simulink model "cart_phase_control"  (R2013b)
settings: Solver=FixedStepDiscrete  StartTime=0.0  StopTime=4  FixedStep=0.000250  MaxStep=0.5  RelTol=1e-3
InitFcn:
  | % Second Order System Parameters
  | wn = 100;   % Natural Frequency (rad/sec)
  | d  = .4;        % Damping Ratio
libraries: xpclib x5, xpcnilib x2, dspmtrx3 x2, powerlib_meascontrol x1, dspadpt3 x1
Description:
  | This model demonstrates three different representations
  | of a 2nd-Order system.
settings Model: ModifiedHistory="05 Feb 2002  Created."  ExtModeTrigMode=oneshot  ExtModeArmWhenConnect=off  BufferReuse=off  Creator=Douglas G. Jones  LastModifiedBy=bzr3
settings DataIOCC: LimitDataPoints=off  SignalLoggingSaveFormat=ModelDataLogs  SaveOutput=off  SignalLogging=off  SaveTime=off
settings OptimizationCC: BlockReduction=off  BooleanDataType=off  OptimizeBlockIOStorage=off  BufferReuse=off  ExpressionFolding=off  ExpressionDepthLimit=2147483647  LocalBlockOutputs=off  InitFltsAndDblsToZero=on
settings DebuggingCC: SaveWithParameterizedLinksMsg=none  SignalResolutionControl=TryResolveAllWithWarning  SolverPrmCheckMsg=none  MultiTaskDSMMsg=warning  MultiTaskCondExecSysMsg=none  FcnCallInpInsideContextMsg=UseLocalSettings  StateNameClashWarn=warning  StrictBusMsg=None
settings HardwareCC: ProdIntDivRoundTo=Zero  ProdEndianess=LittleEndian  ProdHWDeviceType=Generic->32-bit x86 compatible  TargetLongLongMode=on  TargetEndianess=LittleEndian  TargetHWDeviceType=MATLAB Host
settings RTWCC: SystemTargetFile=xpctarget.tlc  TemplateMakefile=xpc_default_tmf  RTWVerbose=off  ProcessScript=xpctarget_make_rtw_hook  IncludeERTFirstTime=on  RTWCompilerOptimization=On
settings TargetCC: TargetFcnLib=ansi_tfl_tmw.mat  CodeReplacementLibrary=XPC_BLAS  IsPILTarget=off  ParMdlRefBuildCompliant=on  ConcurrentExecutionCompliant=on  MatFileLogging=on  EnableShiftOperators=on
settings ConfigurationSet: Description=SimMechanics 2G

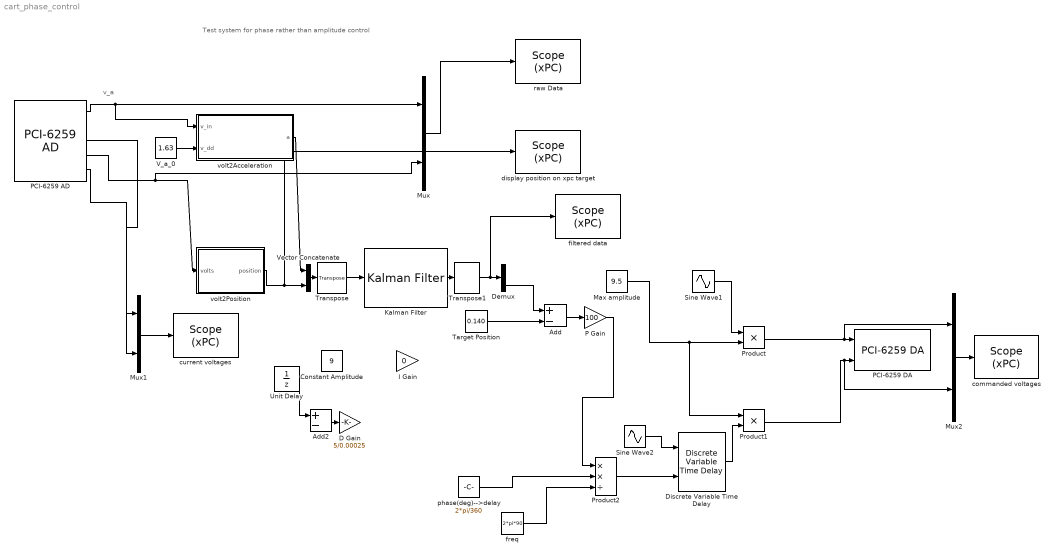
== system cart_phase_control ==
  note: Test system for phase rather than amplitude control
  note: v_a
  Add : Sum  Inputs=+-
  Add2 : Sum  Inputs=+-
  Constant Amplitude : Constant  Value=9
  D Gain : Gain  Gain=5/0.00025
  Demux : Demux  Outputs=2
  Discrete Variable Time Delay : powerlib_meascontrol/Additional Components/Discrete Variable Time Delay  MaxDelay=1  InitialValue=0  Ts=0.00025  DFT=on
  I Gain : Gain  Gain=0
  Kalman Filter : dspadpt3/Kalman Filter  num_targets=1  sourceEnable=Always  isReset=on  X=[0.15;0;0]  P=10*eye(3)  A=[1,2.500000000000000e-04,6.250000000000000e-08;0,1,2.500000000000000e-04;0,0,1]  sourceMeasure=Specify via Dialog  H=[1 0 0; 0 0 1]  Q=0.05*eye(3)  R=[10 0; 0 10]  isOutputEstMeasure=on  isOutputEstState=off  isOutputEstError=off  isOutputPrdMeasure=off  isOutputPrdState=off  isOutputPrdError=off
  Max amplitude : Constant  Value=9.5
  Mux : Mux  Inputs=2
  Mux1 : Mux  Inputs=2
  Mux2 : Mux  Inputs=2
  P Gain : Gain  Gain=100
  PCI-6259 AD : xpcnilib/A//D/M Series/PCI-6259 AD  channel=[1 7 14 16 6]  range=[10]  coupling=[0]  scantime=5e-6  sampletime=0.000250  slot=-1
  PCI-6259 DA : xpcnilib/D//A/M Series/PCI-6259 DA  channel=[1 2]  range=[10]  reset=[1]  initValue=[0]  sampletime=0.00025  slot=-1
  Product : Product  RndMeth=Zero
  Product1 : Product  RndMeth=Zero
  Product2 : Product  Inputs=**/  RndMeth=Zero
  Sine Wave1 : Sin  Frequency=2*pi*90  SampleTime=0
  Sine Wave2 : Sin  Frequency=2*pi*90  Phase=270*pi/180  SampleTime=0
  Target Position : Constant  Value=0.140
  Transpose : dspmtrx3/Transpose  Hermitian=off  overflowFlag=off
  Transpose1 : dspmtrx3/Transpose  Hermitian=off  overflowFlag=off
  Unit Delay : UnitDelay  SampleTime=-1
  V_a_0 : Constant  Value=1.63
  Vector Concatenate : Concatenate  Mode=Multidimensional array  ConcatenateDimension=2
  commanded voltages : xpclib/Misc./Scope (xPC)   scopeno=4  scopetype=Host  autostart=on  viewmode=Graphical redraw  formatstr='%15.6f'  grid=on  ylimits=[0,0]  nosamples=16001  noprepostsamples=0  interleave=1  triggermode=FreeRun  triggersignal=1  trigsignalfromport=off  triggerlevel=0.0  triggerslope=Either  triggerscope=1  triggersample=0  filename=sosLog.dat  mode=Lazy  writesize=512  autorestart=off  dynamicfilemode=off  maxwritefilesize=512*1024^2
  current voltages : xpclib/Misc./Scope (xPC)   scopeno=3  scopetype=Host  autostart=on  viewmode=Graphical redraw  formatstr='%15.6f'  grid=on  ylimits=[0,0]  nosamples=16001  noprepostsamples=0  interleave=1  triggermode=FreeRun  triggersignal=1  trigsignalfromport=off  triggerlevel=0.0  triggerslope=Either  triggerscope=1  triggersample=0  filename=sosLog.dat  mode=Lazy  writesize=512  autorestart=off  dynamicfilemode=off  maxwritefilesize=512*1024^2
  "display position on xpc target " : xpclib/Misc./Scope (xPC)   scopeno=1  scopetype=Target  autostart=on  viewmode=Graphical sliding  formatstr='%15.6f'  grid=on  ylimits=[0,0]  nosamples=16001  noprepostsamples=0  interleave=1  triggermode=FreeRun  triggersignal=1  trigsignalfromport=off  triggerlevel=0.0  triggerslope=Either  triggerscope=1  triggersample=0  filename=sosLog.dat  mode=Lazy  writesize=512  autorestart=off  dynamicfilemode=off  maxwritefilesize=512*1024^2
  filtered data : xpclib/Misc./Scope (xPC)   scopeno=2  scopetype=Host  autostart=on  viewmode=Graphical redraw  formatstr='%15.6f'  grid=on  ylimits=[0,0]  nosamples=16001  noprepostsamples=0  interleave=1  triggermode=FreeRun  triggersignal=1  trigsignalfromport=off  triggerlevel=0.0  triggerslope=Either  triggerscope=1  triggersample=0  filename=sosLog.dat  mode=Lazy  writesize=512  autorestart=off  dynamicfilemode=off  maxwritefilesize=512*1024^2
  freq : Constant  Value=2*pi*90
  phase(deg)-->delay : Constant  Value=2*pi/360
  raw Data : xpclib/Misc./Scope (xPC)   scopeno=5  scopetype=Host  autostart=on  viewmode=Graphical redraw  formatstr='%15.6f'  grid=on  ylimits=[0,0]  nosamples=16001  noprepostsamples=0  interleave=1  triggermode=FreeRun  triggersignal=1  trigsignalfromport=off  triggerlevel=0.0  triggerslope=Either  triggerscope=1  triggersample=0  filename=sosLog.dat  mode=Lazy  writesize=512  autorestart=off  dynamicfilemode=off  maxwritefilesize=512*1024^2
  volt2Acceleration : Subsystem
  "volt2Position " : Subsystem
  wires:
  PCI-6259 AD/1 -> volt2Acceleration/1(v_in), Mux/1
  Mux/1 -> raw Data/1
  Kalman Filter/1 -> Transpose1/1
  Transpose1/1 -> filtered data/1, Demux/1
  Transpose/1 -> Kalman Filter/1
  Vector Concatenate/1 -> Transpose/1
  "volt2Position "/1("position ") -> Vector Concatenate/2, "display position on xpc target "/1
  volt2Acceleration/1(a) -> Vector Concatenate/1
  PCI-6259 AD/4 -> "volt2Position "/1(volts), Mux/2
  PCI-6259 AD/3 -> Mux1/1
  PCI-6259 AD/5 -> Mux1/2
  Mux1/1 -> current voltages/1
  Sine Wave1/1 -> Product/1
  Demux/2 -> Add/1
  Target Position/1 -> Add/2
  Max amplitude/1 -> Product/2, Product1/1
  Add/1 -> P Gain/1
  P Gain/1 -> Product2/1
  V_a_0/1 -> volt2Acceleration/2(v_dd)
  Product/1 -> Mux2/1, PCI-6259 DA/1
  Add2/1 -> D Gain/1
  Unit Delay/1 -> Add2/1
  Mux2/1 -> commanded voltages/1
  Product1/1 -> Mux2/2, PCI-6259 DA/2
  Sine Wave2/1 -> Discrete Variable Time Delay/1
  Discrete Variable Time Delay/1 -> Product1/2
  freq/1 -> Product2/3
  phase(deg)-->delay/1 -> Product2/2
  Product2/1 -> Discrete Variable Time Delay/2

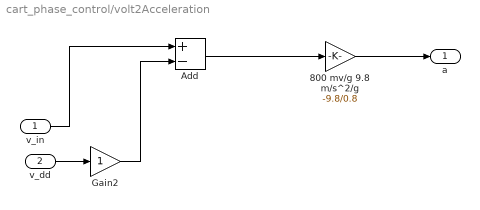
== system cart_phase_control/volt2Acceleration ==
  v_in : Inport
  v_dd : Inport  Port=2
  800 mv/g 9.8 m/s^2/g : Gain  Gain=-9.8/0.8
  Add : Sum  Inputs=+-
  Gain2 : Gain
  a : Outport
  wires:
  v_in/1 -> Add/1
  800 mv/g 9.8 m/s^2/g/1 -> a/1
  Add/1 -> 800 mv/g 9.8 m/s^2/g/1
  v_dd/1 -> Gain2/1
  Gain2/1 -> Add/2

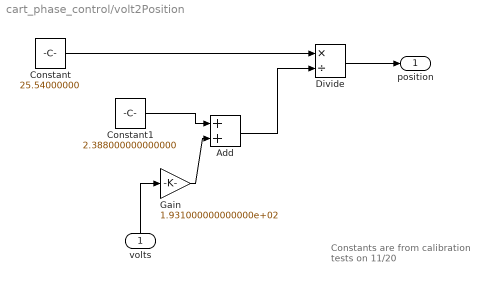
== system cart_phase_control/volt2Position  ==
  note: Constants are from calibration tests on 11/20
  volts : Inport
  Add : Sum
  Constant : Constant  Value=25.54000000
  Constant1 : Constant  Value=2.388000000000000
  Divide : Product  Inputs=*/
  Gain : Gain  Gain=1.931000000000000e+02
  "position " : Outport
  wires:
  volts/1 -> Gain/1
  Constant1/1 -> Add/1
  Gain/1 -> Add/2
  Divide/1 -> "position "/1
  Add/1 -> Divide/2
  Constant/1 -> Divide/1
